simulink model "LaneFollowingWithMonoCameraTestBench"  (R2019b)
settings: Solver=VariableStepAuto  StartTime=0.0  StopTime=scenario.StopTime  RelTol=1e-3
PostLoadFcn:
  | laneFollowingWithMonoCameraSetup
undefined symbols (not defined in the file): assessment, Ts, v_set
libraries: simulink x2
CloseFcn:
  | helperLFMonoCameraCleanUp
settings Model: Creator=The MathWorks, Inc.  LastModifiedBy=senoa95
settings DataIOCC: SaveOutput=off  SaveTime=off  ReturnWorkspaceOutputs=off
settings DebuggingCC: ParameterPrecisionLossMsg=none  PregeneratedLibrarySubsystemCodeDiagnostic=none  ArithmeticOperatorsInVariantConditions=warning
settings HardwareCC: ProdLongLongMode=on
settings SFSimCC: SimUseLocalCustomCode=off
settings RTWCC: RTWUseLocalCustomCode=off
settings ConfigComp: CovScope=ReferencedModels  CovIncludeTopModel=off

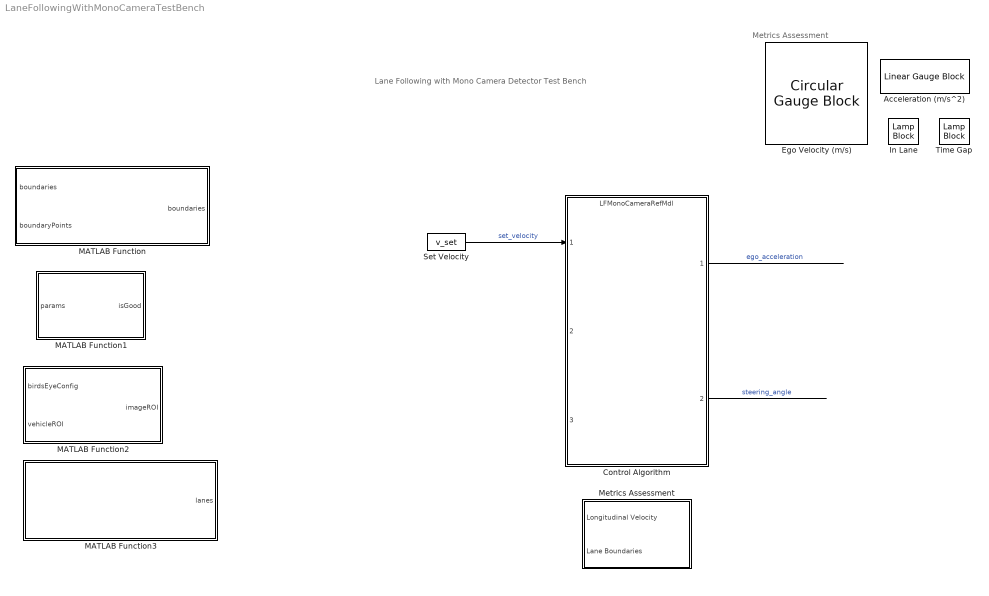
== system LaneFollowingWithMonoCameraTestBench ==
  note: Lane Following with Mono Camera Detector
      | Test Bench
  note: Metrics Assessment
  Acceleration (m/s^2) : LinearGaugeBlock  LabelPosition=Hide  ScaleMin=-6  ScaleMax=6
  Control Algorithm : ModelReference  ModelNameDialog=LFMonoCameraRefMdl.slx  SimulationMode=Normal  CodeInterface=Top model  ModelReferenceVersion=1.758
  Ego Velocity (m/s) : CircularGaugeBlock  LabelPosition=Hide  ScaleMax=50
  In Lane : LampBlock  LabelPosition=Hide
  MATLAB Function : MATLAB Function  TreatAsAtomicUnit=on
  MATLAB Function1 : MATLAB Function  TreatAsAtomicUnit=on
  MATLAB Function2 : MATLAB Function  TreatAsAtomicUnit=on
  MATLAB Function3 : MATLAB Function  TreatAsAtomicUnit=on
  "Metrics Assessment " : Subsystem
  Set Velocity : Constant  Value=v_set  SampleTime=Ts
  Time Gap : LampBlock  LabelPosition=Hide
  wires:
  Control Algorithm/1 -> ?  "ego_acceleration"
  Control Algorithm/2 -> ?  "steering_angle"
  Set Velocity/1 -> Control Algorithm/1  "set_velocity"
  ? -> "Metrics Assessment "/2(Lane Boundaries)  "lane_boundaries"
  ? -> "Metrics Assessment "/1(Longitudinal Velocity), Control Algorithm/2

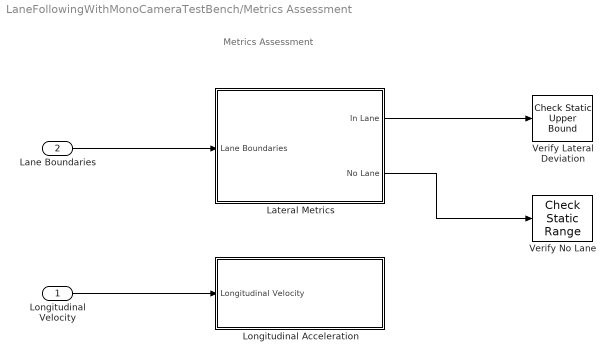
== system LaneFollowingWithMonoCameraTestBench/Metrics Assessment  ==
  note: Metrics Assessment
  Longitudinal Velocity : Inport
  Lane Boundaries : Inport  Port=2
  Lateral Metrics : Subsystem
  Longitudinal Acceleration : Subsystem
  Verify Lateral Deviation : simulink/Model Verification/Check Static  Upper Bound  Description=u <= assessment.LateralDeviationMax  max=assessment.LateralDeviationMax  max_included=on  enabled=on  stopWhenAssertionFail=off  export=off  icon=graphic
      settings: SourceProductName=Simulink  SourceProductBaseCode=SL
      settings: AttributesFormatString=|
      | ---------------------------------------
      | max = %<max>
  Verify No Lane : simulink/Model Verification/Check  Static Range  Description=0 <= u <= 0  max=0  max_included=on  min=0  min_included=on  enabled=on  stopWhenAssertionFail=on  export=off  icon=graphic
      settings: SourceProductName=Simulink  SourceProductBaseCode=SL
  wires:
  Lateral Metrics/1(In Lane) -> Verify Lateral Deviation/1
  Longitudinal Velocity/1 -> Longitudinal Acceleration/1(Longitudinal Velocity)
  Lane Boundaries/1 -> Lateral Metrics/1(Lane Boundaries)
  Lateral Metrics/2(No Lane) -> Verify No Lane/1

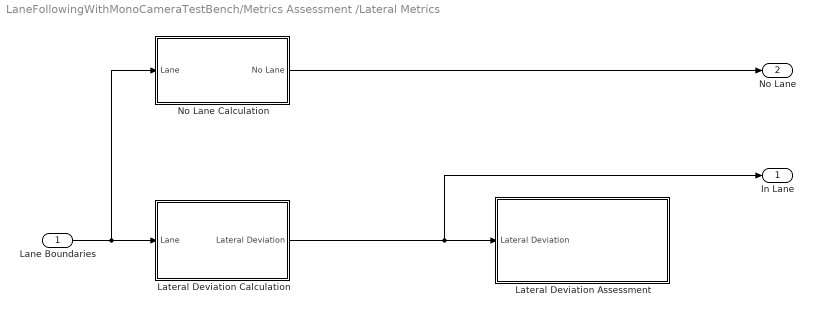
== system LaneFollowingWithMonoCameraTestBench/Metrics Assessment /Lateral Metrics ==
  Lane Boundaries : Inport
  Lateral Deviation Assessment : Subsystem
  Lateral Deviation Calculation : Subsystem
  No Lane Calculation : Subsystem
  In Lane : Outport  VectorParamsAs1DForOutWhenUnconnected=off
  No Lane : Outport  Port=2
  wires:
  Lateral Deviation Calculation/1(Lateral Deviation) -> In Lane/1, Lateral Deviation Assessment/1(Lateral Deviation)
  No Lane Calculation/1(No Lane) -> No Lane/1
  Lane Boundaries/1 -> No Lane Calculation/1(Lane), Lateral Deviation Calculation/1(Lane)

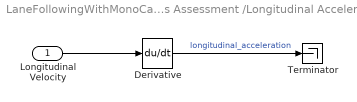
== system LaneFollowingWithMonoCameraTestBench/Metrics Assessment /Longitudinal Acceleration ==
  Longitudinal Velocity : Inport
  Derivative : Derivative
  Terminator : Terminator
  wires:
  Derivative/1 -> Terminator/1  "longitudinal_acceleration"
  Longitudinal Velocity/1 -> Derivative/1

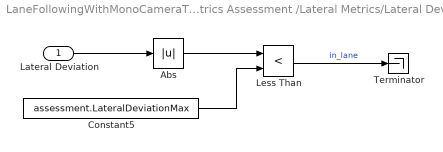
== system LaneFollowingWithMonoCameraTestBench/Metrics Assessment /Lateral Metrics/Lateral Deviation Assessment ==
  Lateral Deviation : Inport
  Abs : Abs
  Constant5 : Constant  Value=assessment.LateralDeviationMax
  Less Than : RelationalOperator  Operator=<  OutDataTypeStr=boolean  RndMeth=Simplest
  Terminator : Terminator
  wires:
  Constant5/1 -> Less Than/2
  Abs/1 -> Less Than/1
  Less Than/1 -> Terminator/1  "in_lane"
  Lateral Deviation/1 -> Abs/1

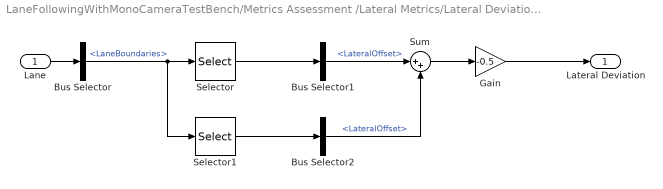
== system LaneFollowingWithMonoCameraTestBench/Metrics Assessment /Lateral Metrics/Lateral Deviation Calculation ==
  Lane : Inport
  Bus Selector : BusSelector  OutputSignals=LaneBoundaries
  Bus Selector1 : BusSelector  OutputSignals=LateralOffset
  Bus Selector2 : BusSelector  OutputSignals=LateralOffset
  Gain : Gain  Gain=-0.5
  Selector : Selector  InputPortWidth=2  IndexOptions=Index vector (dialog)  Indices=1  OutputSizes=1
  Selector1 : Selector  InputPortWidth=2  IndexOptions=Index vector (dialog)  Indices=2  OutputSizes=1
  Sum : Sum  Inputs=|++
  Lateral Deviation : Outport
  wires:
  Lane/1 -> Bus Selector/1
  Selector/1 -> Bus Selector1/1
  Bus Selector2/1 -> Sum/2  "<LateralOffset>"
  Selector1/1 -> Bus Selector2/1
  Sum/1 -> Gain/1
  Bus Selector1/1 -> Sum/1  "<LateralOffset>"
  Bus Selector/1 -> Selector1/1, Selector/1  "<LaneBoundaries>"
  Gain/1 -> Lateral Deviation/1

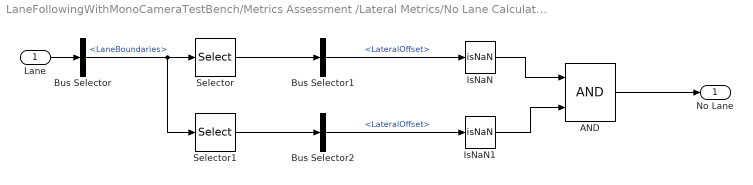
== system LaneFollowingWithMonoCameraTestBench/Metrics Assessment /Lateral Metrics/No Lane Calculation ==
  Lane : Inport
  AND : Logic  IconShape=distinctive  AllPortsSameDT=off  OutDataTypeStr=boolean
  Bus Selector : BusSelector  OutputSignals=LaneBoundaries
  Bus Selector1 : BusSelector  OutputSignals=LateralOffset
  Bus Selector2 : BusSelector  OutputSignals=LateralOffset
  IsNaN : RelationalOperator  Operator=isNaN  OutDataTypeStr=boolean  RndMeth=Simplest
  IsNaN1 : RelationalOperator  Operator=isNaN  OutDataTypeStr=boolean  RndMeth=Simplest
  Selector : Selector  InputPortWidth=2  IndexOptions=Index vector (dialog)  Indices=1  OutputSizes=1
  Selector1 : Selector  InputPortWidth=2  IndexOptions=Index vector (dialog)  Indices=2  OutputSizes=1
  No Lane : Outport
  wires:
  Selector1/1 -> Bus Selector2/1
  Bus Selector/1 -> Selector1/1, Selector/1  "<LaneBoundaries>"
  Selector/1 -> Bus Selector1/1
  Lane/1 -> Bus Selector/1
  Bus Selector1/1 -> IsNaN/1  "<LateralOffset>"
  Bus Selector2/1 -> IsNaN1/1  "<LateralOffset>"
  IsNaN/1 -> AND/1
  IsNaN1/1 -> AND/2
  AND/1 -> No Lane/1

== matlab function LaneFollowingWithMonoCameraTestBench/MATLAB Function1 ==
  data: params input; isGood output
function isGood = validateBoundaryFcn(params)

if ~isempty(params)
    a = params(1);
    
    % Reject any curve with a small 'a' coefficient, which makes it highly
    % curved.
    isGood = abs(a) < 0.003; % a from ax^2+bx+c
else
    isGood = false;
end
end

== matlab function LaneFollowingWithMonoCameraTestBench/MATLAB Function ==
  data: boundaries input; boundaries output; boundaryPoints input
function boundaries = classifyLaneTypes(boundaries, boundaryPoints)

for bInd = 1 : numel(boundaries)
    vehiclePoints = boundaryPoints{bInd};
    % Sort by x
    vehiclePoints = sortrows(vehiclePoints, 1);
    
    xVehicle = vehiclePoints(:,1);
    xVehicleUnique = unique(xVehicle);
    
    % Dashed vs solid
    xdiff  = diff(xVehicleUnique);
    % Sufficiently large threshold to remove spaces between points of a
    % solid line, but not large enough to remove spaces between dashes
    xdifft = mean(xdiff) + 3*std(xdiff);
    largeGaps = xdiff(xdiff > xdifft);
    
    % Safe default
    boundaries(bInd).BoundaryType= LaneBoundaryType.Solid;
    if largeGaps>2
        % Ideally, these gaps should be consistent, but you cannot rely
        % on that unless you know that the ROI extent includes at least 3 dashes.
        boundaries(bInd).BoundaryType = LaneBoundaryType.Dashed;
    end
end

end

== matlab function LaneFollowingWithMonoCameraTestBench/MATLAB Function2 ==
  data: birdsEyeConfig input; imageROI output; vehicleROI input
function imageROI = vehicleToImageROI(birdsEyeConfig, vehicleROI)

vehicleROI = double(vehicleROI);

loc2 = abs(vehicleToImage(birdsEyeConfig, [vehicleROI(2) vehicleROI(4)]));
loc1 = abs(vehicleToImage(birdsEyeConfig, [vehicleROI(1) vehicleROI(4)]));
loc4 =     vehicleToImage(birdsEyeConfig, [vehicleROI(1) vehicleROI(4)]);
loc3 =     vehicleToImage(birdsEyeConfig, [vehicleROI(1) vehicleROI(3)]);

[minRoiX, maxRoiX, minRoiY, maxRoiY] = deal(loc4(1), loc3(1), loc2(2), loc1(2));

imageROI = round([minRoiX, maxRoiX, minRoiY, maxRoiY]);

end

== matlab function LaneFollowingWithMonoCameraTestBench/MATLAB Function3 ==
  data: lanes output
function lanes = detect_lanes()
%% initialize camara intrinsics
% focalLength = cameraParams.FocalLength;
% principalPoint = cameraParams.PrincipalPoint;
% imageSize = cameraParams.ImageSize;
focalLength = [637.8722,637.0641];
principalPoint = [323.5977,239.8220];
imageSize      = [480, 640];  
camIntrinsics = cameraIntrinsics(focalLength, principalPoint, imageSize);

%% determine camera sensor placement
height = 0.3;    % mounting height in meters from the ground
pitch  = 0;        % pitch of the camera in degrees
sensor = monoCamera(camIntrinsics, height, 'Pitch', pitch);
%% initialize matlab ros node
if robotics.ros.internal.Global.isNodeActive == 0
    rosinit
end

for i = 1:10000
%% subscribe to compressed camera image
cam_topic = '/usb_cam/image_raw/compressed';
sub = rossubscriber(cam_topic);
msg = sub.receive;
frame = msg.readImage;

%% specify lane detection parameters
distAheadOfSensor = 15; % in meters, as previously specified in monoCamera height input
spaceToOneSide    = 5;  % all other distance quantities are also in meters
bottomOffset      = 0;

outView   = [bottomOffset, distAheadOfSensor, -spaceToOneSide, spaceToOneSide]; % [xmin, xmax, ymin, ymax]
imageSize = [NaN, 250]; % output image width in pixels; height is chosen automatically to preserve units per pixel ratio

%% transform image
birdsEyeConfig = birdsEyeView(sensor, outView, imageSize);

birdsEyeImage = transformImage(birdsEyeConfig, frame);

% Convert to grayscale
birdsEyeImage = rgb2gray(birdsEyeImage);

% Lane marker segmentation ROI in world units
vehicleROI = outView - [0, 0, -0.85, 0.85]; % look 3 meters to left and right, and 4 meters ahead of the sensor
approxLaneMarkerWidthVehicle = 0.1; % 25 centimeters

%% detect lane 
% Detect lane features
laneSensitivity = 0.2;
birdsEyeViewBW = segmentLaneMarkerRidge(birdsEyeImage, birdsEyeConfig, approxLaneMarkerWidthVehicle,...
    'ROI', vehicleROI, 'Sensitivity', laneSensitivity);

[imageX, imageY] = find(birdsEyeViewBW);
xyBoundaryPoints = imageToVehicle(birdsEyeConfig, [imageY, imageX]);

maxLanes      = 2; % look for maximum of two lane markers
boundaryWidth = 3*approxLaneMarkerWidthVehicle; % expand boundary width

[frame, boundaryPoints] = findCubicLaneBoundaries(xyBoundaryPoints,boundaryWidth, ...
    'MaxNumBoundaries', maxLanes, 'validateBoundaryFcn', @validateBoundaryFcn);

%% filter lanes
% Establish criteria for rejecting boundaries based on their length
maxPossibleXLength = diff(vehicleROI(1:2));
minXLength         = maxPossibleXLength * 0.60; % establish a threshold

% Reject short boundaries
isOfMinLength = arrayfun(@(b)diff(b.XExtent) > minXLength, frame);
frame    = frame(isOfMinLength);

%% convert lanes to vehicle frame
% To compute the maximum strength, assume all image pixels within the ROI
% are lane candidate points
birdsImageROI = vehicleToImageROI(birdsEyeConfig, vehicleROI);
[laneImageX,laneImageY] = meshgrid(birdsImageROI(1):birdsImageROI(2),birdsImageROI(3):birdsImageROI(4));

% Convert the image points to vehicle points
vehiclePoints = imageToVehicle(birdsEyeConfig,[laneImageX(:),laneImageY(:)]);

% Find the maximum number of unique x-axis locations possible for any lane
% boundary
maxPointsInOneLane = numel(unique(vehiclePoints(:,1)));

% Set the maximum length of a lane boundary to the ROI length
maxLaneLength = diff(vehicleROI(1:2));

% Compute the maximum possible lane strength for this image size/ROI size
% specification
maxStrength   = maxPointsInOneLane/maxLaneLength;

% Reject weak boundaries
isStrong      = [frame.Strength] > 0.4*maxStrength;
frame    = frame(isStrong);

frame = classifyLaneTypes(frame, boundaryPoints);

% Locate two ego lanes if they are present
xOffset    = 0;   %  0 meters from the sensor
distanceToBoundaries  = frame.computeBoundaryModel(xOffset);

% Find candidate ego boundaries
leftEgoBoundaryIndex  = [];
rightEgoBoundaryIndex = [];
minLDistance = min(distanceToBoundaries(distanceToBoundaries>0));
minRDistance = max(distanceToBoundaries(distanceToBoundaries<=0));
if ~isempty(minLDistance)
    leftEgoBoundaryIndex  = distanceToBoundaries == minLDistance;
end
if ~isempty(minRDistance)
    rightEgoBoundaryIndex = distanceToBoundaries == minRDistance;
end

leftEgoBoundary       = frame(leftEgoBoundaryIndex);
rightEgoBoundary      = frame(rightEgoBoundaryIndex);

%% display left and right lane clothoid parameters

if ~isempty(leftEgoBoundary)
    disp('left lane params')
    disp(leftEgoBoundary.Parameters)
end

if ~isempty(rightEgoBoundary)
    disp('right lane params')
    disp(rightEgoBoundary.Parameters)
end


end
